simulink model "Spring_model"  (R2021b)
settings: Solver=VariableStepAuto  StartTime=0.0  StopTime=90  MaxStep=0.001  RelTol=1e-3  AbsTol=1e-3  EnableMultiTasking=on
PreLoadFcn:
  | m = 3.600;     % kg
  | k = 400;    % N/m
  | b = 10;      % Ns/m
  | x0=1; %m
undefined symbols (not defined in the file): rMax, rMin
CloseFcn:
  | try,close(h1_ssc_mass_spring_damper_sl),end
  | clear h1_ssc_mass_spring_damper_sl
  | 
  | clear simlog_ssc_mass_spring_damper_sl
  | clear logsout_ssc_mass_spring_damper_sl
Description:
  | Mass-Spring-Damper in Simulink(R) and Simscape(TM)
settings Model: Creator=The MathWorks, Inc.  LastModifiedBy=jacks
settings SolverCC: AutoScaleAbsTol=off  AlgebraicLoopSolver=TrustRegion
settings DataIOCC: SaveFormat=Array  ReturnWorkspaceOutputs=off  SignalLoggingName=logsout_ssc_mass_spring_damper_sl
settings OptimizationCC: LifeSpan=inf
settings DebuggingCC: SolverPrmCheckMsg=warning  AllowSymbolicDim=off  PregeneratedLibrarySubsystemCodeDiagnostic=none  SFUnexpectedBacktrackingDiag=warning  SFNoUnconditionalDefaultTransitionDiag=warning  SFExecutionAtInitializationDiag=none  SFMachineParentedDataDiag=warning  ArithmeticOperatorsInVariantConditions=warning
settings HardwareCC: ProdBitPerPointer=32  ProdBitPerSizeT=32  ProdBitPerPtrDiffT=32  ProdLargestAtomicFloat=None  ProdIntDivRoundTo=Undefined  ProdEndianess=Unspecified  ProdWordSize=32  ProdHWDeviceType=32-bit Generic
settings ModelReferenceCC: PropagateSignalLabelsOutOfModel=off
settings SFSimCC: SimUseLocalCustomCode=off  CustomCodeUndefinedFunction=UseInterfaceOnly
settings RTWCC: RTWUseLocalCustomCode=off
settings CodeAppCC: StateflowObjectComments=on
settings GRTTargetCC: TargetLangStandard=C89/C90 (ANSI)
settings ConfigComp: CovMetricSettings=dw  CovSaveCumulativeToWorkspaceVar=on  CovSaveSingleToWorkspaceVar=on  CovExternalEMLEnable=off  CovSFcnEnable=off
settings SimscapeCC: SimscapeLogType=all  SimscapeLogSimulationStatistics=on  SimscapeLogName=simlog_ssc_mass_spring_damper_sl  SimscapeLogDataHistory=10000

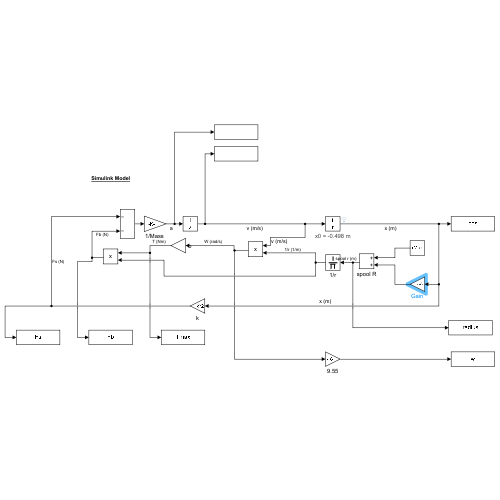
[thumbnail: Simulink's stored preview of the top-level diagram]
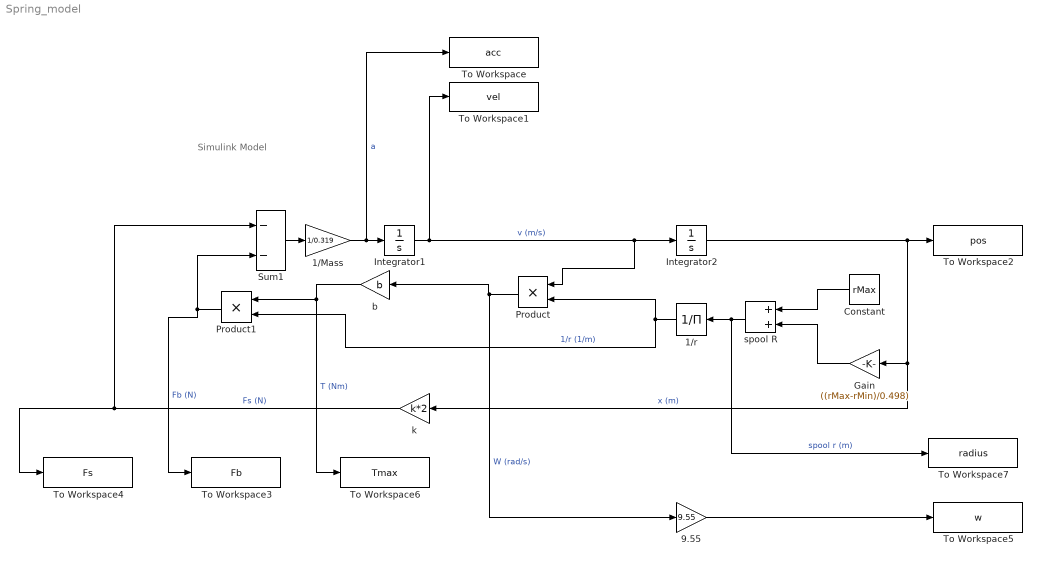
== system Spring_model ==
  note: Simulink Model
  "1/Mass " : Gain  Gain=1/0.319  SaturateOnIntegerOverflow=on  OutDataTypeStr=Inherit: Same as input  ParamDataTypeStr=Inherit: Same as input
  1/r : Product  Inputs=/
  9.55 : Gain  Gain=9.55
  Constant : Constant  Value=rMax
  Gain : Gain  Gain=((rMax-rMin)/0.498)
  Integrator1 : Integrator
  Integrator2 : Integrator  InitialCondition=-0.498
      settings: AttributesFormatString=x0 = %<InitialCondition> m
  Product : Product
  Product1 : Product
  Sum1 : Sum  Inputs=--  InputSameDT=on  SaturateOnIntegerOverflow=on  OutDataTypeStr=Inherit: Same as first input
  To Workspace : ToWorkspace  VariableName=acc  SampleTime=-1
  To Workspace1 : ToWorkspace  VariableName=vel  SampleTime=-1
  To Workspace2 : ToWorkspace  VariableName=pos  SampleTime=-1
  To Workspace3 : ToWorkspace  VariableName=Fb  SampleTime=-1
  To Workspace4 : ToWorkspace  VariableName=Fs  SampleTime=-1
  To Workspace5 : ToWorkspace  VariableName=w  SampleTime=-1
  To Workspace6 : ToWorkspace  VariableName=Tmax  SampleTime=-1
  To Workspace7 : ToWorkspace  VariableName=radius  SampleTime=-1
  b : Gain  Gain=b
  k : Gain  Gain=k*2  SaturateOnIntegerOverflow=on  OutDataTypeStr=Inherit: Same as input  ParamDataTypeStr=Inherit: Same as input
  spool R : Sum
  wires:
  "1/Mass "/1 -> To Workspace/1, Integrator1/1  "a"
  Sum1/1 -> "1/Mass "/1
  k/1 -> Sum1/1, To Workspace4/1  "Fs (N)"
  Integrator2/1 -> Gain/1, k/1, To Workspace2/1  "x (m)"
  Integrator1/1 -> Integrator2/1, Product/1, To Workspace1/1  "v (m/s)"
  b/1 -> Product1/1, To Workspace6/1  "T (Nm)"
  Gain/1 -> spool R/2
  Constant/1 -> spool R/1
  spool R/1 -> To Workspace7/1, 1/r/1  "spool r (m)"
  1/r/1 -> Product1/2, Product/2  "1/r (1/m)"
  Product/1 -> 9.55/1, b/1  "W (rad/s)"
  Product1/1 -> Sum1/2, To Workspace3/1  "Fb (N)"
  9.55/1 -> To Workspace5/1
